simulink model "v2b_test"  (R2018a)
settings: Solver=FixedStepAuto  StartTime=0.0  StopTime=10.0  FixedStep=1  MaxStep=1  RelTol=1e-3
PreLoadFcn:
  | mybus = Simulink.Bus();
  | elem_ = Simulink.BusElement();
  | 
  | elem_.Name  = 'dblElem';
  | elem_.DataType = 'double';
  | elem_.Dimensions = 2;
  | mybus.Elements(1) = elem_;
  | 
  | elem_.Name  = 'intElem';
  | elem_.DataType = 'int32';
  | elem_.Dimensions = [1 3];
  | mybus.Elements(2) = elem_;
  | 
  | elem_.Name  = 'boolElem';
  | elem_.DataType = 'boolean';
  | elem_.Dimensions = 1;
  | mybus.Elements(3) = elem_;
  | 
  | clear elem_
libraries: v2b_lib x1
settings Model: Creator=thomas  LastModifiedBy=thomas
settings DataIOCC: SaveOutput=off  SignalLogging=off  DSMLogging=off  SaveTime=off
settings HardwareCC: ProdBitPerLong=64  ProdHWDeviceType=Intel->x86-64 (Linux 64)
settings RTWCC: GenerateReport=on  LaunchReport=on
settings CodeAppCC: SimulinkBlockComments=off
settings GRTTargetCC: MatFileLogging=off  SupportNonFinite=off

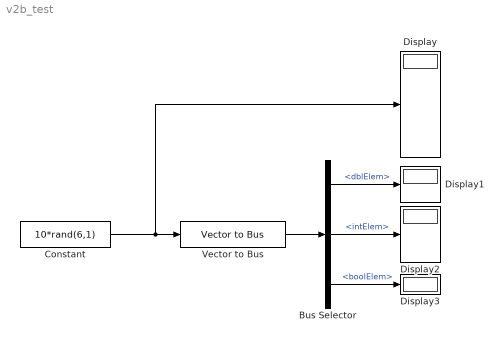
== system v2b_test ==
  Bus Selector : BusSelector  OutputSignals=dblElem,intElem,boolElem
  Constant : Constant  Value=10*rand(6,1)  SampleTime=1
  Display{,1..3} (4 alike) : Display
  Vector to Bus : v2b_lib/Vector to Bus  busName=Bus: mybus
  wires:
  Constant/1 -> Display/1, Vector to Bus/1
  Vector to Bus/1 -> Bus Selector/1
  Bus Selector/1 -> Display1/1  "<dblElem>"
  Bus Selector/2 -> Display2/1  "<intElem>"
  Bus Selector/3 -> Display3/1  "<boolElem>"
